simulink model "Q1F_LinearXQ1Q2"  (R2015b)
settings: Solver=VariableStepAuto  StartTime=0.0  StopTime=100  RelTol=1e-3
values from neighbouring files (symbols this model uses):
  A = [ 0, 1,                  0, 0,                      0, 0 ... (first row only)    [Q1E.m]    (also in Q1F_Init_Models_Overall.m = [ 0, 1,               0,     0,              0, 0; Q1F_Init_Models_x.m = [ 0, 1,               0,     0,              0, 0; Q1F_Init_Models_xQ1Q2.m = [ 0, 1,               0,     0,              0, 0; Q1F_Init_Models_xQ2.m = [ 0, 1,               0,     0,              0, 0)
  AxQ1Q2_obs = [A-LxQ1Q2*CxQ1Q2]    [Q1F_Init_Models_Overall.m]    (also in Q1F_Init_Models_xQ1Q2.m)
  B = [  0 ... (first row only)    [Q1E.m]    (also in Q1F_Init_Models_Overall.m = [ 0; Q1F_Init_Models_x.m = [ 0; Q1F_Init_Models_xQ1Q2.m = [ 0; Q1F_Init_Models_xQ2.m = [ 0)
  BxQ1Q2_obs = [B LxQ1Q2]    [Q1F_Init_Models_Overall.m]    (also in Q1F_Init_Models_xQ1Q2.m)
  C_all = eye(6)    [Q1F_Init_Models_Overall.m]    (also in Q1F_Init_Models_x.m; Q1F_Init_Models_xQ1Q2.m; Q1F_Init_Models_xQ2.m; Q1G_Init_Model.m)
  CxQ1Q2 = [1 0 0 0 0 0 ... (first row only)    [Q1F_Init_Models_Overall.m]    (also in Q1F_Init_Models_xQ1Q2.m)
  D = zeros(6,1)    [Q1E.m]    (also in Q1F_Init_Models_Overall.m; Q1F_Init_Models_x.m; Q1F_Init_Models_xQ1Q2.m; Q1F_Init_Models_xQ2.m)
  DxQ1Q2_obs = [0 0 0 0; 0 0 0 0;0 0 0 0;0 0 0 0;0 0 0 0;0 0 0 0]    [Q1F_Init_Models_Overall.m]    (also in Q1F_Init_Models_xQ1Q2.m)
  X_0_l = [0 0 X_0(3)*pi/180 X_0(4)*pi/180 X_0(5)*pi/180 X_0(6)*pi/180]'    [Q1E.m]    (also in Q1F_Init_Models_Overall.m = [X_0(1) X_0(2) X_0(3)*pi/180 X_0(4)*pi/180 X_0(5)*pi/180 X_0; Q1F_Init_Models_x.m = [X_0(1) X_0(2) X_0(3)*pi/180 X_0(4)*pi/180 X_0(5)*pi/180 X_0; Q1F_Init_Models_xQ1Q2.m = [X_0(1) X_0(2) X_0(3)*pi/180 X_0(4)*pi/180 X_0(5)*pi/180 X_0; Q1F_Init_Models_xQ2.m = [X_0(1) X_0(2) X_0(3)*pi/180 X_0(4)*pi/180 X_0(5)*pi/180 X_0)
  X_0_xQ1Q2_obs = [0 0 0 0 0 0]    [Q1F_Init_Models_Overall.m]    (also in Q1F_Init_Models_xQ1Q2.m)
undefined symbols (not defined in the file or in its folder): K
settings Model: Creator=Chirag  LastModifiedBy=ANKUR

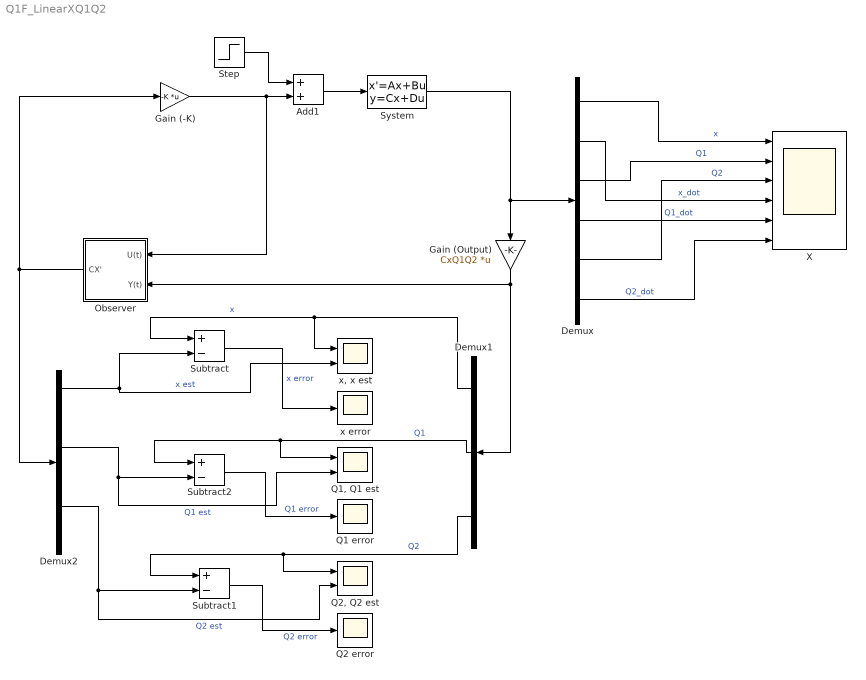
== system Q1F_LinearXQ1Q2 ==
  Add1 : Sum
  Demux : Demux  Outputs=6
  Demux1 : Demux  Outputs=3
  Demux2 : Demux  Outputs=6
  Gain (-K) : Gain  Gain=-K  Multiplication=Matrix(K*u) (u vector)
  Gain (Output) : Gain  Gain=CxQ1Q2  Multiplication=Matrix(K*u) (u vector)
  Observer : Subsystem
  Q1 error : Scope
  "Q1, Q1 est" : Scope  NumInputPorts=2
  Q2 error : Scope
  "Q2, Q2 est" : Scope  NumInputPorts=2
  Step : Step  Time=0  SampleTime=0
  Subtract : Sum  Inputs=+-
  Subtract1 : Sum  Inputs=+-
  Subtract2 : Sum  Inputs=+-
  System : StateSpace  A=A  B=B  C=C_all  D=D  X0=X_0_l
  X : Scope  NumInputPorts=6
  x error : Scope
  "x, x est" : Scope  NumInputPorts=2
  wires:
  System/1 -> Gain (Output)/1, Demux/1
  Gain (-K)/1 -> Add1/2, Observer/1(U(t))
  Observer/1(CX') -> Demux2/1, Gain (-K)/1
  Gain (Output)/1 -> Demux1/1, Observer/2(Y(t))
  Add1/1 -> System/1
  Step/1 -> Add1/1
  Demux/1 -> X/1  "x"
  Demux/3 -> X/2  "Q1"
  Demux/5 -> X/3  "Q2"
  Demux/2 -> X/4  "x_dot"
  Demux/4 -> X/5  "Q1_dot"
  Demux/6 -> X/6  "Q2_dot"
  Demux1/1 -> "x, x est"/1, Subtract/1  "x"
  Demux2/1 -> "x, x est"/2, Subtract/2  "x est"
  Subtract/1 -> x error/1  "x error"
  Demux1/3 -> "Q2, Q2 est"/1, Subtract1/1  "Q2"
  Demux2/5 -> "Q2, Q2 est"/2, Subtract1/2  "Q2 est"
  Subtract1/1 -> Q2 error/1  "Q2 error"
  Demux1/2 -> "Q1, Q1 est"/1, Subtract2/1  "Q1"
  Demux2/3 -> "Q1, Q1 est"/2, Subtract2/2  "Q1 est"
  Subtract2/1 -> Q1 error/1  "Q1 error"

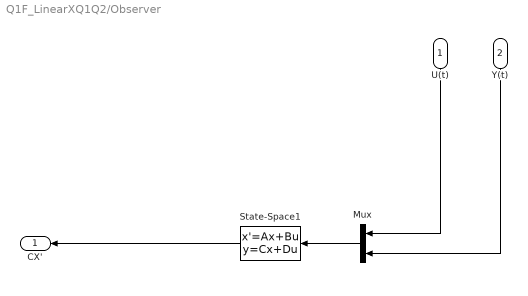
== system Q1F_LinearXQ1Q2/Observer ==
  U(t) : Inport
  Y(t) : Inport  Port=2
  Mux : Mux  Inputs=2
  State-Space1 : StateSpace  A=AxQ1Q2_obs  B=BxQ1Q2_obs  C=C_all  D=DxQ1Q2_obs  X0=X_0_xQ1Q2_obs
  CX' : Outport
  wires:
  State-Space1/1 -> CX'/1
  Mux/1 -> State-Space1/1
  U(t)/1 -> Mux/1
  Y(t)/1 -> Mux/2
